simulink model "benchmark_ivan_PIANN"  (R2024b)
settings: Solver=FixedStepAuto  StartTime=0.0  StopTime=14  FixedStep=0.0001  RelTol=1e-5  AbsTol=1e-8  EnableMultiTasking=on
values from neighbouring files (symbols this model uses):
  b1 = csvread('./DAE_ANN/ANN/Biases/30_04_21/lstm_ann_pi_standard_fix_noSo4_rnn_1__100_16_b_3.csv')    [init_PI_ann.m]    (also in init_PI_ann_hier.m = csvread('./DAE_ANN/ANN/Biases/12_05_21/lstm_ann_pi_standard_; init_PI_ann_hier_v2.m = csvread('./DAE_ANN/ANN/Biases/12_05_21/lstm_ann_pi_standard_; init_PI_ann_lab.m = csvread('./DAE_ANN/ANN/Biases/12_05_21/lstm_ann_pi_standard_)
  b2 = csvread('./DAE_ANN/ANN/Biases/30_04_21/lstm_ann_pi_standard_fix_noSo4_rnn_1__100_16_b_3.csv')    [init_PI_ann.m]    (also in init_PI_ann_hier.m = csvread('./DAE_ANN/ANN/Biases/12_05_21/lstm_ann_pi_standard_; init_PI_ann_hier_v2.m = csvread('./DAE_ANN/ANN/Biases/12_05_21/lstm_ann_pi_standard_; init_PI_ann_lab.m = csvread('./DAE_ANN/ANN/Biases/12_05_21/lstm_ann_pi_standard_)
  b_last = csvread('./DAE_ANN/ANN/Biases/12_05_21/lstm_ann_pi_standard_fix_noSo4_last__100_1_b_2.csv')'    [init_PI_ann_hier.m]    (also in init_PI_ann_hier_v2.m; init_PI_ann_lab.m)
  b_out = csvread('./DAE_ANN/ANN/Biases/30_04_21/lstm_ann_pi_standard_fix_noSo4_final__100_16_b_3.csv')    [init_PI_ann.m]    (also in init_PI_ann_hier.m = csvread('./DAE_ANN/ANN/Biases/12_05_21/lstm_ann_pi_standard_; init_PI_ann_hier_v2.m = csvread('./DAE_ANN/ANN/Biases/12_05_21/lstm_ann_pi_standard_; init_PI_ann_lab.m = csvread('./DAE_ANN/ANN/Biases/12_05_21/lstm_ann_pi_standard_)
  ic_sw_Kla = 145*ones(n_sw,1)    [init_PI_ann.m]    (also in init_PI_ann_hier.m; init_PI_ann_hier_v2.m; init_PI_ann_lab.m)
  ic_sw_Snh4 = 6*ones(n_sw,1)    [init_PI_ann.m]    (also in init_PI_ann_hier.m; init_PI_ann_hier_v2.m; init_PI_ann_lab.m)
  ic_sw_Sno4 = 8*ones(n_sw,1)    [init_PI_ann.m]    (also in init_PI_ann_hier.m; init_PI_ann_hier_v2.m; init_PI_ann_lab.m)
  ic_sw_So4 = 3*ones(n_sw,1)    [init_PI_ann.m]    (also in init_PI_ann_hier.m; init_PI_ann_hier_v2.m; init_PI_ann_lab.m)
  ic_sw_So5 = 2*ones(n_sw,1)    [init_PI_ann.m]    (also in init_PI_ann_hier.m; init_PI_ann_hier_v2.m; init_PI_ann_lab.m)
  KLa5_max = 360    [sensorinit.m]
  max_Q4 = 100000    [sensorinit.m]
  max_SNH4 = 20    [sensorinit.m]
  max_SNO2 = 20    [sensorinit.m]
  max_SNO4 = 20    [sensorinit.m]
  max_SO4 = 10    [sensorinit.m]
  max_SO5 = 10    [sensorinit.m]    (also in setup_Prac5.m = 5)
  max_TSS4 = 10000    [sensorinit.m]
  mean_scaler_dir = csvread('./DAE_ANN/ANN/Scalers/30_04_21_lstm_ann_pi_standard_fix_noSo4/mean_scaler_lstm_ann_pi_standard_fix_noSo4.csv')    [init_PI_ann.m]    (also in init_PI_ann_hier.m = csvread('./DAE_ANN/ANN/Scalers/12_05_21_lstm_ann_pi_standard; init_PI_ann_hier_v2.m = csvread('./DAE_ANN/ANN/Scalers/12_05_21_lstm_ann_pi_standard; setup_Prac5.m = [(Q/k)^2, 1.9756, 0.0000, 0]')
  mean_scaler_dir_out = csvread('./DAE_ANN/ANN/Scalers/30_04_21_lstm_ann_pi_standard_fix_noSo4/mean_scaler_lstm_ann_pi_standard_fix_noSo4_out.csv')    [init_PI_ann.m]    (also in init_PI_ann_hier.m = csvread('./DAE_ANN/ANN/Scalers/12_05_21_lstm_ann_pi_standard; init_PI_ann_hier_v2.m = csvread('./DAE_ANN/ANN/Scalers/12_05_21_lstm_ann_pi_standard; setup_Prac5.m = 0)
  min_Q4 = 0    [sensorinit.m]
  min_SNH4 = 0    [sensorinit.m]
  min_SNO2 = 0    [sensorinit.m]
  min_SNO4 = 0    [sensorinit.m]
  min_SO5 = 0    [sensorinit.m]
  min_TSS4 = 0    [sensorinit.m]
  n_layers = 1    [init_PI_ann.m]    (also in init_PI_ann_hier.m; init_PI_ann_hier_v2.m; init_PI_ann_lab.m)
  n_sw = 16    [init_PI_ann.m]    (also in init_PI_ann_hier.m = 1; init_PI_ann_hier_v2.m = 1; init_PI_ann_lab.m = 1)
  n_sw_inverse = 16    [init_PI_ann.m]    (also in init_PI_ann_hier.m = 1; init_PI_ann_hier_v2.m = 1; init_PI_ann_lab.m = 1)
  noiseseed_Q4 = 1    [sensorinit.m]
  noiseseed_SNH4 = 2    [sensorinit.m]
  noiseseed_SNO2 = 2    [sensorinit.m]
  noiseseed_SNO4 = 2    [sensorinit.m]
  noiseseed_SO4 = 2    [sensorinit.m]
  noiseseed_SO5 = 1    [sensorinit.m]
  noiseseed_TSS4 = 1    [sensorinit.m]
  noisesource_Q4 = 1    [sensorinit.m]
  noisesource_SNH4 = 1    [sensorinit.m]
  noisesource_SNO2 = 1    [sensorinit.m]
  noisesource_SNO4 = 1    [sensorinit.m]
  noisesource_SO4 = 1    [sensorinit.m]
  noisesource_SO5 = 1    [sensorinit.m]
  noisesource_TSS4 = 1    [sensorinit.m]
  Qin0 = 18446    [states.mat]
  Qintr = 12141.8126939    [states.mat]
  Qintr_max = 5*Qin0    [sensorinit.m]
  Qintrawstate = 114243.527362    [states.mat]
  Qintrintstate = -116205.765277    [states.mat]
  SETTLERINIT = [12.5979803087 18.2981709885 29.6744598765 68.7829340492 352.293497132 353.981663079 351.499035887 351.323930185 355.679725774 6417.21684783 30 30 ... (80 elements, 1x80)]    [states.mat]
  Sno_mean = 1    [run_bsm1_PIANN_variable.m]
  SO5awstate = 469.399689831    [states.mat]
  SO5intstate = -450.70071346    [states.mat]
  SO5ref = 2    [run_bsm1_PIANN.m]    (also in run_bsm1_PIANN_variable.m)
  So_mean = 2    [run_bsm1_PIANN_variable.m]    (also in setup_Prac5.m = 0.2)
  std_Q4 = 0.025    [sensorinit.m]
  std_scaler_dir = csvread('./DAE_ANN/ANN/Scalers/30_04_21_lstm_ann_pi_standard_fix_noSo4/std_scaler_lstm_ann_pi_standard_fix_noSo4.csv')    [init_PI_ann.m]    (also in init_PI_ann_hier.m = csvread('./DAE_ANN/ANN/Scalers/12_05_21_lstm_ann_pi_standard; init_PI_ann_hier_v2.m = csvread('./DAE_ANN/ANN/Scalers/12_05_21_lstm_ann_pi_standard; setup_Prac5.m = [1, 0.7579, 0.05, 1]')
  std_scaler_dir_out = csvread('./DAE_ANN/ANN/Scalers/30_04_21_lstm_ann_pi_standard_fix_noSo4/std_scaler_lstm_ann_pi_standard_fix_noSo4_out.csv')    [init_PI_ann.m]    (also in init_PI_ann_hier.m = csvread('./DAE_ANN/ANN/Scalers/12_05_21_lstm_ann_pi_standard; init_PI_ann_hier_v2.m = csvread('./DAE_ANN/ANN/Scalers/12_05_21_lstm_ann_pi_standard; setup_Prac5.m = 1)
  std_SNH4 = 0.025    [sensorinit.m]
  std_SNO2 = 0.025    [sensorinit.m]
  std_SO4 = 0.025    [sensorinit.m]
  std_SO5 = 0.025    [sensorinit.m]
  std_TSS4 = 0.025    [sensorinit.m]
  T = 6.5201    [setup_Prac5.m]
  t_init = 7e-3    (= 0.007)    [run_bsm1.m]    (also in run_bsm1_PIANN_variable.m = 0.05)
  T_KLa5 = T90_KLa5/(24*60)/3.89    (= 0.000714081690945)    [sensorinit.m]
  T_Q4 = T90_Q4/(24*60)/3.89    (= 0.000178520422736)    [sensorinit.m]
  t_simulink = 1/96    (= 0.0104166666667)    [run_bsm1.m]    (also in run_bsm1_PIANN.m = -1; run_bsm1_PIANN_variable.m = 0; setup_Prac5.m = 0)
  T_SNH4 = T90_SNH4/(24*60)/11.7724    (= 0.000589891988417)    [sensorinit.m]
  T_SNO2 = T90_SNO2/(24*60)/11.7724    (= 0.000589891988417)    [sensorinit.m]
  T_SNO4 = T90_SNO4/(24*60)/11.7724    (= 0.000589891988417)    [sensorinit.m]
  T_SO5 = T90_SO5/(24*60)/3.89    (= 0.000178520422736)    [sensorinit.m]
  T_TSS4 = T90_TSS4/(24*60)/3.89    (= 0.000178520422736)    [sensorinit.m]
  t_zero_order = -1    [run_bsm1_PIANN.m]    (also in run_bsm1_PIANN_variable.m)
  u1 = csvread('./DAE_ANN/ANN/Weights/30_04_21/lstm_ann_pi_standard_fix_noSo4_rnn_1__100_16_U_3.csv')    [init_PI_ann.m]    (also in init_PI_ann_hier.m = csvread('./DAE_ANN/ANN/Weights/12_05_21/lstm_ann_pi_standard; init_PI_ann_hier_v2.m = csvread('./DAE_ANN/ANN/Weights/12_05_21/lstm_ann_pi_standard)
  u2 = csvread('./DAE_ANN/ANN/Weights/30_04_21/lstm_ann_pi_standard_fix_noSo4_rnn_1__100_16_U_3.csv')    [init_PI_ann.m]    (also in init_PI_ann_hier.m = csvread('./DAE_ANN/ANN/Weights/12_05_21/lstm_ann_pi_standard; init_PI_ann_hier_v2.m = csvread('./DAE_ANN/ANN/Weights/12_05_21/lstm_ann_pi_standard)
  useideal_KLa5 = 0    [run_bsm1.m]    (also in run_bsm1_PIANN.m = 1; run_bsm1_PIANN_variable.m = 1; sensorinit.m)
  useideal_Q4 = 1    [run_bsm1_PIANN.m]    (also in run_bsm1_PIANN_variable.m; sensorinit.m = 0)
  useideal_SNH4 = 0    [run_bsm1.m]    (also in run_bsm1_PIANN.m = 1; run_bsm1_PIANN_variable.m = 1; sensorinit.m)
  useideal_SNO2 = 1    [run_bsm1_PIANN.m]    (also in run_bsm1_PIANN_variable.m; sensorinit.m = 0)
  useideal_SNO4 = 0    [run_bsm1.m]    (also in run_bsm1_PIANN.m = 1; run_bsm1_PIANN_variable.m = 1; sensorinit.m)
  useideal_SO4 = 0    [run_bsm1.m]    (also in run_bsm1_PIANN.m = 1; run_bsm1_PIANN_variable.m = 1; sensorinit.m)
  useideal_SO5 = 0    [run_bsm1.m]    (also in run_bsm1_PIANN.m = 1; run_bsm1_PIANN_variable.m = 1; sensorinit.m)
  useideal_TSS4 = 1    [run_bsm1_PIANN.m]    (also in run_bsm1_PIANN_variable.m; sensorinit.m = 0)
  usenoise_Q4 = 0    [run_bsm1_PIANN.m]    (also in run_bsm1_PIANN_variable.m; sensorinit.m = 1)
  usenoise_SNH4 = 1    [run_bsm1.m]    (also in run_bsm1_PIANN.m = 0; run_bsm1_PIANN_variable.m = 0; sensorinit.m)
  usenoise_SNO2 = 0    [run_bsm1_PIANN.m]    (also in run_bsm1_PIANN_variable.m; sensorinit.m = 1)
  usenoise_SNO4 = 1    [run_bsm1.m]    (also in run_bsm1_PIANN.m = 0; run_bsm1_PIANN_variable.m = 0; sensorinit.m)
  usenoise_SO4 = 1    [run_bsm1.m]    (also in run_bsm1_PIANN.m = 0; run_bsm1_PIANN_variable.m = 0; sensorinit.m)
  usenoise_SO5 = 1    [run_bsm1.m]    (also in run_bsm1_PIANN.m = 0; run_bsm1_PIANN_variable.m = 0; sensorinit.m)
  usenoise_TSS4 = 0    [run_bsm1_PIANN.m]    (also in run_bsm1_PIANN_variable.m; sensorinit.m = 1)
  w1 = csvread('./DAE_ANN/ANN/Weights/30_04_21/lstm_ann_pi_standard_fix_noSo4_rnn_1__100_16_W_3.csv')    [init_PI_ann.m]    (also in init_PI_ann_hier.m = csvread('./DAE_ANN/ANN/Weights/12_05_21/lstm_ann_pi_standard; init_PI_ann_hier_v2.m = csvread('./DAE_ANN/ANN/Weights/12_05_21/lstm_ann_pi_standard; init_PI_ann_lab.m = csvread('./DAE_ANN/ANN/Weights/12_05_21/lstm_ann_pi_standard)
  w2 = csvread('./DAE_ANN/ANN/Weights/30_04_21/lstm_ann_pi_standard_fix_noSo4_rnn_1__100_16_W_3.csv')    [init_PI_ann.m]    (also in init_PI_ann_hier.m = csvread('./DAE_ANN/ANN/Weights/12_05_21/lstm_ann_pi_standard; init_PI_ann_hier_v2.m = csvread('./DAE_ANN/ANN/Weights/12_05_21/lstm_ann_pi_standard; init_PI_ann_lab.m = csvread('./DAE_ANN/ANN/Weights/12_05_21/lstm_ann_pi_standard)
  w_last = csvread('./DAE_ANN/ANN/Weights/12_05_21/lstm_ann_pi_standard_fix_noSo4_last__100_1_W_2.csv')    [init_PI_ann_hier.m]    (also in init_PI_ann_hier_v2.m; init_PI_ann_lab.m)
  w_out = csvread('./DAE_ANN/ANN/Weights/30_04_21/lstm_ann_pi_standard_fix_noSo4_final__100_16_W_3.csv')    [init_PI_ann.m]    (also in init_PI_ann_hier.m = csvread('./DAE_ANN/ANN/Weights/12_05_21/lstm_ann_pi_standard; init_PI_ann_hier_v2.m = csvread('./DAE_ANN/ANN/Weights/12_05_21/lstm_ann_pi_standard; init_PI_ann_lab.m = csvread('./DAE_ANN/ANN/Weights/12_05_21/lstm_ann_pi_standard)
  XINIT1 = [30 3.2250440682 1132.84750814 98.0848162551 2520.32093658 147.34360098 454.498440184 0.006943357113 3.54207658602 12.0720627837 1.35151294762 6.05742445882 ... (15 elements, 1x15)]    [states.mat]
  XINIT2 = [30 1.63865407136 1124.24951453 88.653599068 2501.35826654 146.001740625 452.094465666 5.17099136584e-05 1.14245691502 13.0383387996 0.796493225193 5.70045637375 ... (15 elements, 1x15)]    [states.mat]
  XINIT3 = [30 1.20592174915 1120.58961418 67.1871738861 2499.94635325 146.547839977 452.007772249 1.74081325353 6.26492922945 8.40116301472 0.827753486834 4.51387309735 ... (15 elements, 1x15)]    [states.mat]
  XINIT4 = [30 0.96656120797 1121.66055561 52.7833355811 2504.32671079 147.644975737 453.890499756 2.40137566232 11.073804945 3.99279026202 0.746788866766 3.70339113264 ... (15 elements, 1x15)]    [states.mat]
  XINIT5 = [30 0.803395489358 1124.12455116 43.2595495328 2508.23031357 148.499403125 456.322790044 2.11978031988 14.1356901459 1.15379834533 0.659650038761 3.15951382084 ... (15 elements, 1x15)]    [states.mat]
  XINITDELAY = [1466770.04249 1266021.87556 55799754.9774 5815431.95778 123179806.598 7263098.80912 22318785.5012 62039.7687555 416609.519268 588047.303413 143684.636473 343270.852984 ... (15 elements, 1x15)]    [states.mat]
undefined symbols (not defined in the file or in its folder): b_bottle, b_decoder_1, b_decoder_2, b_encoder_1, b_encoder_2, b_final, b_out_dae, carb1, carb2, carb3, carb4, carb5, DIM, Kfeedforward, KLa1, KLa2, KLa3, KLa4, KLa5offset, KQintr, KSO5, LAYER, magnitude, mean_scaler_dae, mean_scaler_dae_out, MODELTYPE, PAR1, PAR2, PAR3, PAR4, PAR5, Qffref, Qintroffset, QintrT, SETTLERPAR, SNO2ref, SOSAT1, SOSAT2, SOSAT3, SOSAT4, SOSAT5, std_scaler_dae, std_scaler_dae_out, TiQintr, TiSO5, TtQintr, TtSO5, u_decoder_1, u_decoder_2, u_encoder_1, u_encoder_2, useantiwindupQintr, useantiwindupSO5, VOL1, VOL2, VOL3, VOL4, VOL5, w_bottle, w_decoder_1 ... (+5)
libraries: dspindex x33
(part 2 of 4)

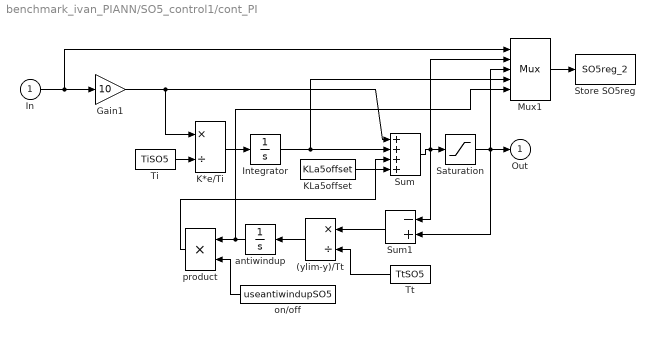
== system benchmark_ivan_PIANN/SO5_control1/cont_PI ==
  In : Inport
  (ylim-y)/Tt : Product  Inputs=*/  InputSameDT=on  SaturateOnIntegerOverflow=on  OutDataTypeStr=Inherit: Same as first input
  Gain1 : Gain  Gain=10  SaturateOnIntegerOverflow=on  OutDataTypeStr=Inherit: Same as input  ParamDataTypeStr=Inherit: Same as input
  Integrator : Integrator  InitialCondition=SO5intstate
  K*e/Ti : Product  Inputs=*/  InputSameDT=on  SaturateOnIntegerOverflow=on  OutDataTypeStr=Inherit: Same as first input
  KLa5offset : Constant  Value=KLa5offset
  Mux1 : Mux  Inputs=5
  Saturation : Saturate  UpperLimit=KLa5_max  LowerLimit=0
  Store SO5reg : ToWorkspace  VariableName=SO5reg_2  SampleTime=-1
  Sum : Sum  Inputs=++++  InputSameDT=on  SaturateOnIntegerOverflow=on  OutDataTypeStr=Inherit: Same as first input
  Sum1 : Sum  Inputs=-+  InputSameDT=on  SaturateOnIntegerOverflow=on  OutDataTypeStr=Inherit: Same as first input
  Ti : Constant  Value=TiSO5
  Tt : Constant  Value=TtSO5
  antiwindup : Integrator  InitialCondition=SO5awstate
  on/off : Constant  Value=useantiwindupSO5
  product : Product  Inputs=**  InputSameDT=on  SaturateOnIntegerOverflow=on  OutDataTypeStr=Inherit: Same as first input
  Out : Outport  VectorParamsAs1DForOutWhenUnconnected=off
  wires:
  product/1 -> Sum/3
  on/off/1 -> product/2
  K*e/Ti/1 -> Integrator/1
  Ti/1 -> K*e/Ti/2
  Gain1/1 -> Sum/1, K*e/Ti/1
  Sum1/1 -> (ylim-y)/Tt/1
  Tt/1 -> (ylim-y)/Tt/2
  (ylim-y)/Tt/1 -> antiwindup/1
  Sum/1 -> Saturation/1, Sum1/1, Mux1/2
  Saturation/1 -> Out/1, Sum1/2, Mux1/3
  Mux1/1 -> Store SO5reg/1
  Integrator/1 -> Sum/2, Mux1/4
  antiwindup/1 -> product/1, Mux1/5
  KLa5offset/1 -> Sum/4
  In/1 -> Gain1/1, Mux1/1

== system benchmark_ivan_PIANN/SO5_control_paper/Filter_Prediction ==
  Kla5 : Inport
  So5_noise : Inport  Port=2
  Measurements_1 : Inport  Port=3
  DAE_MLP1 : Subsystem  Commented=on
  DAE_MLP2 : Subsystem  Commented=on
  DAE_MLP3 : Subsystem
  DAE_lstm : Subsystem  Commented=on
  Direct Prediction LSTM4 : Subsystem
  Inverse Data : Subsystem
  Terminator : Terminator  Commented=on
  To Workspace5 : ToWorkspace  VariableName=clean_data  SampleTime=1/96
      settings: Save2DSignal=2-D array (concatenate along first dimension)
  So5_clean : Outport
  wires:
  DAE_MLP3/1(Output) -> Direct Prediction LSTM4/2(meas1), To Workspace5/1
  Inverse Data/1(Snh4) -> DAE_MLP3/1(Snh4)
  Inverse Data/2(TSS4) -> DAE_MLP3/2(TSS4)
  Inverse Data/3(Q4) -> DAE_MLP3/3(Q4)
  Kla5/1 -> Direct Prediction LSTM4/1(kla1)
  Measurements_1/1 -> Inverse Data/1(y_n1)
  Direct Prediction LSTM4/1(y_n) -> So5_clean/1
  So5_noise/1 -> DAE_MLP3/4("So5_noise ")

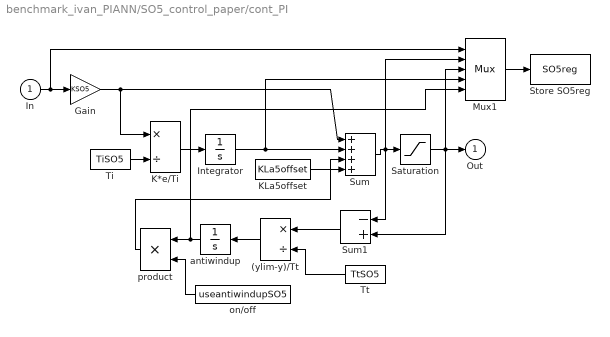
== system benchmark_ivan_PIANN/SO5_control_paper/cont_PI ==
  In : Inport
  (ylim-y)/Tt : Product  Inputs=*/  InputSameDT=on  SaturateOnIntegerOverflow=on  OutDataTypeStr=Inherit: Same as first input
  Gain : Gain  Gain=KSO5  SaturateOnIntegerOverflow=on  OutDataTypeStr=Inherit: Same as input  ParamDataTypeStr=Inherit: Same as input
  Integrator : Integrator  InitialCondition=SO5intstate
  K*e/Ti : Product  Inputs=*/  InputSameDT=on  SaturateOnIntegerOverflow=on  OutDataTypeStr=Inherit: Same as first input
  KLa5offset : Constant  Value=KLa5offset
  Mux1 : Mux  Inputs=5
  Saturation : Saturate  UpperLimit=KLa5_max  LowerLimit=0
  Store SO5reg : ToWorkspace  VariableName=SO5reg  SampleTime=-1
  Sum : Sum  Inputs=++++  InputSameDT=on  SaturateOnIntegerOverflow=on  OutDataTypeStr=Inherit: Same as first input
  Sum1 : Sum  Inputs=-+  InputSameDT=on  SaturateOnIntegerOverflow=on  OutDataTypeStr=Inherit: Same as first input
  Ti : Constant  Value=TiSO5
  Tt : Constant  Value=TtSO5
  antiwindup : Integrator  InitialCondition=SO5awstate
  on/off : Constant  Value=useantiwindupSO5
  product : Product  Inputs=**  InputSameDT=on  SaturateOnIntegerOverflow=on  OutDataTypeStr=Inherit: Same as first input
  Out : Outport  VectorParamsAs1DForOutWhenUnconnected=off
  wires:
  product/1 -> Sum/3
  on/off/1 -> product/2
  In/1 -> Mux1/1, Gain/1
  K*e/Ti/1 -> Integrator/1
  Ti/1 -> K*e/Ti/2
  Gain/1 -> Sum/1, K*e/Ti/1
  Sum1/1 -> (ylim-y)/Tt/1
  Tt/1 -> (ylim-y)/Tt/2
  (ylim-y)/Tt/1 -> antiwindup/1
  Sum/1 -> Saturation/1, Sum1/1, Mux1/2
  Saturation/1 -> Out/1, Sum1/2, Mux1/3
  Mux1/1 -> Store SO5reg/1
  Integrator/1 -> Sum/2, Mux1/4
  antiwindup/1 -> product/1, Mux1/5
  KLa5offset/1 -> Sum/4

== system benchmark_ivan_PIANN/Direct Prediction 2 LSTM SO1/Data Preprocesing Direct/Normalizer1 ==
  Data Input : Inport
  Normalization Values : MATLAB Function  TreatAsAtomicUnit=on
  Data Normalized : Outport  VectorParamsAs1DForOutWhenUnconnected=off
  wires:
  Data Input/1 -> Normalization Values/1(data_input)
  Normalization Values/1(data_norm) -> Data Normalized/1

== system benchmark_ivan_PIANN/Direct Prediction 2 LSTM SO1/Sliding Window/Sliding Window Buffer So1 ==
  In1 : Inport
  Buffer1 : Buffer  N=16  V=15
  Reshape : Reshape
  Zero-Order Hold : ZeroOrderHold  SampleTime=1/96
  Out1 : Outport
  wires:
  Zero-Order Hold/1 -> Buffer1/1
  In1/1 -> Zero-Order Hold/1
  Reshape/1 -> Out1/1
  Buffer1/1 -> Reshape/1

== system benchmark_ivan_PIANN/Direct Prediction 2 LSTM SO1/Sliding Window/Sliding Window Buffer So2 ==
  In1 : Inport
  Buffer1 : Buffer  N=16  V=15
  Reshape : Reshape
  Zero-Order Hold : ZeroOrderHold  SampleTime=1/96
  Out1 : Outport
  wires:
  Zero-Order Hold/1 -> Buffer1/1
  In1/1 -> Zero-Order Hold/1
  Reshape/1 -> Out1/1
  Buffer1/1 -> Reshape/1

== system benchmark_ivan_PIANN/Direct Prediction 2 LSTM SO1/Sliding Window/Sliding Window Buffer So3 ==
  In1 : Inport
  Buffer1 : Buffer  N=16  V=15
  Reshape : Reshape
  Zero-Order Hold : ZeroOrderHold  SampleTime=-1
  Out1 : Outport
  wires:
  Zero-Order Hold/1 -> Buffer1/1
  In1/1 -> Zero-Order Hold/1
  Reshape/1 -> Out1/1
  Buffer1/1 -> Reshape/1

== system benchmark_ivan_PIANN/Direct Prediction 2 LSTM SO1/Sliding Window/Sliding Window Buffer So4 ==
  In1 : Inport
  Buffer1 : Buffer  N=16  V=15
  Reshape : Reshape
  Zero-Order Hold : ZeroOrderHold  SampleTime=1/96
  Out1 : Outport
  wires:
  Zero-Order Hold/1 -> Buffer1/1
  In1/1 -> Zero-Order Hold/1
  Reshape/1 -> Out1/1
  Buffer1/1 -> Reshape/1

== system benchmark_ivan_PIANN/Direct Prediction LSTM3/Data Preprocesing Direct/Normalizer1 ==
  Data Input : Inport
  Normalization Values : MATLAB Function  TreatAsAtomicUnit=on
  Data Normalized : Outport  VectorParamsAs1DForOutWhenUnconnected=off
  wires:
  Normalization Values/1(data_norm) -> Data Normalized/1
  Data Input/1 -> Normalization Values/1(data_input)

== system benchmark_ivan_PIANN/Direct Prediction LSTM3/Sliding Window/Sliding Window Buffer So1 ==
  In1 : Inport
  Buffer1 : Buffer  N=16  V=15
  Reshape : Reshape
  Zero-Order Hold : ZeroOrderHold  SampleTime=1/96
  Out1 : Outport
  wires:
  Buffer1/1 -> Reshape/1
  Reshape/1 -> Out1/1
  In1/1 -> Zero-Order Hold/1
  Zero-Order Hold/1 -> Buffer1/1

== system benchmark_ivan_PIANN/Direct Prediction LSTM3/Sliding Window/Sliding Window Buffer So2 ==
  In1 : Inport
  Buffer1 : Buffer  N=16  V=15
  Reshape : Reshape
  Zero-Order Hold : ZeroOrderHold  SampleTime=1/96
  Out1 : Outport
  wires:
  Buffer1/1 -> Reshape/1
  Reshape/1 -> Out1/1
  In1/1 -> Zero-Order Hold/1
  Zero-Order Hold/1 -> Buffer1/1

== system benchmark_ivan_PIANN/Direct Prediction LSTM3/Sliding Window/Sliding Window Buffer So3 ==
  In1 : Inport
  Buffer1 : Buffer  N=16  V=15
  Reshape : Reshape
  Zero-Order Hold : ZeroOrderHold  SampleTime=-1
  Out1 : Outport
  wires:
  Buffer1/1 -> Reshape/1
  Reshape/1 -> Out1/1
  In1/1 -> Zero-Order Hold/1
  Zero-Order Hold/1 -> Buffer1/1

== system benchmark_ivan_PIANN/Direct Prediction LSTM3/Sliding Window/Sliding Window Buffer So4 ==
  In1 : Inport
  Buffer1 : Buffer  N=16  V=15
  Reshape : Reshape
  Zero-Order Hold : ZeroOrderHold  SampleTime=1/96
  Out1 : Outport
  wires:
  Buffer1/1 -> Reshape/1
  Reshape/1 -> Out1/1
  In1/1 -> Zero-Order Hold/1
  Zero-Order Hold/1 -> Buffer1/1

== system benchmark_ivan_PIANN/Direct Prediction LSTM3/Sliding Window/Sliding Window1 ==
  ref1 : Inport
  Delay : Delay  DelayLength=1  InitialCondition=0  SampleTime=t_simulink
  Flip : DSPFlip
  IC : InitialCondition  Value=zeros(16,1)
  Mux : Mux  Inputs=2
  Variable Selector : dspindex/Variable Selector  NumInputs=1  rowsOrCols=Rows  IdxMode=Fixed  Elements=1:15  ZerOneIdxMode=One-based  errmode=Clip Index  FillMode=on  FillValues=0
  Out : Outport
  wires:
  IC/1 -> Variable Selector/1
  Delay/1 -> IC/1
  ref1/1 -> Mux/1
  Variable Selector/1 -> Mux/2
  Flip/1 -> Out/1
  Mux/1 -> Delay/1, Flip/1

== system benchmark_ivan_PIANN/Direct Prediction LSTM3/Sliding Window/Sliding Window2 ==
  data : Inport
  Delay : Delay  DelayLength=1  InitialCondition=0  SampleTime=t_simulink
  Flip : DSPFlip
  IC : InitialCondition  Value=zeros(16,1)
  Mux : Mux  Inputs=2
  Variable Selector : dspindex/Variable Selector  NumInputs=1  rowsOrCols=Rows  IdxMode=Fixed  Elements=1:15  ZerOneIdxMode=One-based  errmode=Clip Index  FillMode=on  FillValues=0
  Out : Outport
  wires:
  IC/1 -> Variable Selector/1
  Delay/1 -> IC/1
  data/1 -> Mux/1
  Variable Selector/1 -> Mux/2
  Flip/1 -> Out/1
  Mux/1 -> Delay/1, Flip/1

== system benchmark_ivan_PIANN/Direct Prediction LSTM3/Sliding Window/Sliding Window3 ==
  ref : Inport
  Delay : Delay  DelayLength=1  InitialCondition=0  SampleTime=t_simulink
  Flip : DSPFlip
  IC : InitialCondition  Value=zeros(16,1)
  Mux : Mux  Inputs=2
  Variable Selector : dspindex/Variable Selector  NumInputs=1  rowsOrCols=Rows  IdxMode=Fixed  Elements=1:15  ZerOneIdxMode=One-based  errmode=Clip Index  FillMode=on  FillValues=0
  Out : Outport
  wires:
  IC/1 -> Variable Selector/1
  Delay/1 -> IC/1
  ref/1 -> Mux/1
  Variable Selector/1 -> Mux/2
  Flip/1 -> Out/1
  Mux/1 -> Delay/1, Flip/1

== system benchmark_ivan_PIANN/Direct Prediction LSTM3/Sliding Window/Sliding Window4 ==
  delayed : Inport
  Delay : Delay  DelayLength=1  InitialCondition=0  SampleTime=t_simulink
  Flip : DSPFlip
  IC : InitialCondition  Value=zeros(16,1)
  Mux : Mux  Inputs=2
  Variable Selector : dspindex/Variable Selector  NumInputs=1  rowsOrCols=Rows  IdxMode=Fixed  Elements=1:15  ZerOneIdxMode=One-based  errmode=Clip Index  FillMode=on  FillValues=0
  Out : Outport
  wires:
  IC/1 -> Variable Selector/1
  Delay/1 -> IC/1
  delayed/1 -> Mux/1
  Variable Selector/1 -> Mux/2
  Flip/1 -> Out/1
  Mux/1 -> Delay/1, Flip/1

== system benchmark_ivan_PIANN/Direct Prediction LSTM3/Sliding Window/Sliding Window6 ==
  ref1 : Inport
  Delay : Delay  DelayLength=1  InitialCondition=0  SampleTime=t_simulink
  Flip : DSPFlip
  IC : InitialCondition  Value=zeros(16,1)
  Mux : Mux  Inputs=2
  Variable Selector : dspindex/Variable Selector  NumInputs=1  rowsOrCols=Rows  IdxMode=Fixed  Elements=1:15  ZerOneIdxMode=One-based  errmode=Clip Index  FillMode=on  FillValues=0
  Out : Outport
  wires:
  IC/1 -> Variable Selector/1
  Delay/1 -> IC/1
  ref1/1 -> Mux/1
  Variable Selector/1 -> Mux/2
  Flip/1 -> Out/1
  Mux/1 -> Delay/1, Flip/1

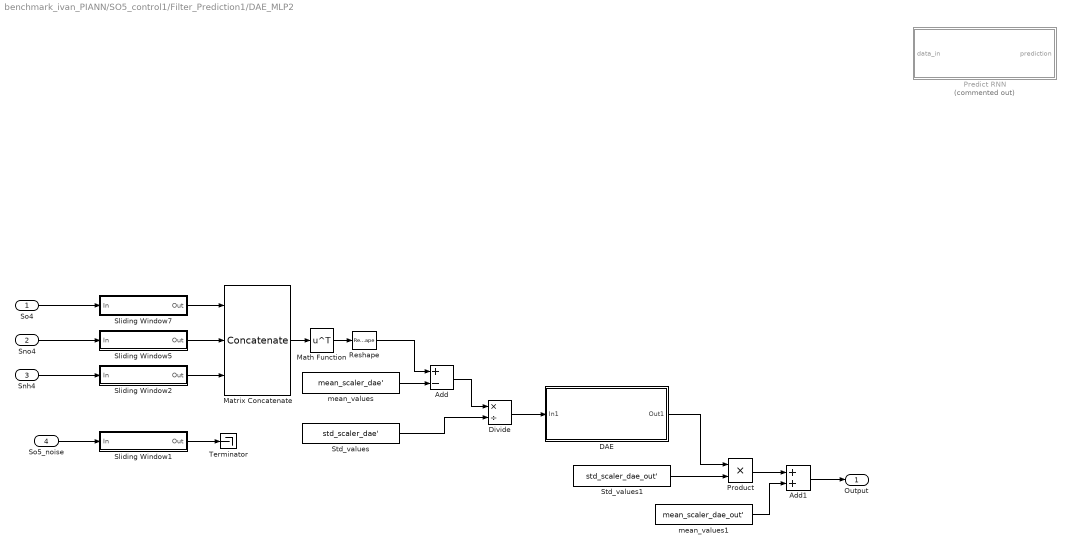
== system benchmark_ivan_PIANN/SO5_control1/Filter_Prediction1/DAE_MLP2 ==
  So4 : Inport
  Sno4 : Inport  Port=2
  Snh4 : Inport  Port=3
  "So5_noise " : Inport  Port=4
  Add : Sum  Inputs=+-
  Add1 : Sum
  DAE : Subsystem
  Divide : Product  Inputs=*/
  Math Function : Math  Operator=transpose  SignedPower=on
  Matrix Concatenate : Concatenate  NumInputs=3  Mode=Multidimensional array  ConcatenateDimension=2
  Predict RNN : MATLAB Function  Commented=on  TreatAsAtomicUnit=on
  Product : Product
  Reshape : Reshape  OutputDimensionality=Row vector (2-D)
  Sliding Window1 : Subsystem
  Sliding Window2 : Subsystem
  Sliding Window5 : Subsystem
  Sliding Window7 : Subsystem
  Std_values : Constant  Value=std_scaler_dae'  VectorParams1D=off
  Std_values1 : Constant  Value=std_scaler_dae_out'  VectorParams1D=off
  Terminator : Terminator
  mean_values : Constant  Value=mean_scaler_dae'  VectorParams1D=off
  mean_values1 : Constant  Value=mean_scaler_dae_out'  VectorParams1D=off
  Output : Outport  VectorParamsAs1DForOutWhenUnconnected=off
  wires:
  Add1/1 -> Output/1
  Sliding Window7/1(Out) -> Matrix Concatenate/1
  Math Function/1 -> Reshape/1
  Matrix Concatenate/1 -> Math Function/1
  Sliding Window1/1(Out) -> Terminator/1
  "So5_noise "/1 -> Sliding Window1/1(In)
  Sliding Window5/1(Out) -> Matrix Concatenate/2
  Sliding Window2/1(Out) -> Matrix Concatenate/3
  Sno4/1 -> Sliding Window5/1(In)
  So4/1 -> Sliding Window7/1(In)
  Snh4/1 -> Sliding Window2/1(In)
  Add/1 -> Divide/1
  Std_values/1 -> Divide/2
  mean_values/1 -> Add/2
  Reshape/1 -> Add/1
  Divide/1 -> DAE/1(In1)
  DAE/1(Out1) -> Product/1
  Std_values1/1 -> Product/2
  Product/1 -> Add1/1
  mean_values1/1 -> Add1/2

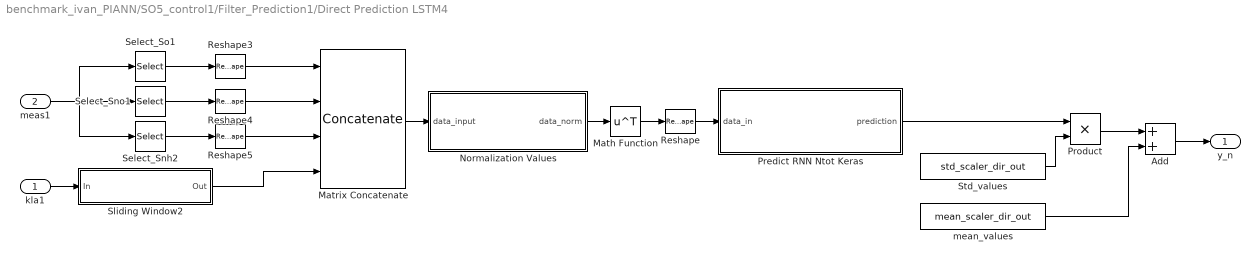
== system benchmark_ivan_PIANN/SO5_control1/Filter_Prediction1/Direct Prediction LSTM4 ==
  kla1 : Inport
  meas1 : Inport  Port=2
  Add : Sum
  Math Function : Math  Operator=transpose  SignedPower=on
  Matrix Concatenate : Concatenate  NumInputs=4  Mode=Multidimensional array  ConcatenateDimension=2
  Normalization Values : MATLAB Function  TreatAsAtomicUnit=on
  Predict RNN Ntot Keras : MATLAB Function  TreatAsAtomicUnit=on
  Product : Product
  Reshape : Reshape  OutputDimensionality=Row vector (2-D)
  Reshape3 : Reshape
  Reshape4 : Reshape
  Reshape5 : Reshape
  Select_Snh2 : Selector  NumberOfDimensions=2  InputPortWidth=4  IndexOptions=Index vector (dialog),Index vector (dialog)  Indices=1,[3:3:48]  OutputSizes=1,1
  Select_Sno1 : Selector  NumberOfDimensions=2  InputPortWidth=4  IndexOptions=Index vector (dialog),Index vector (dialog)  Indices=1,[2:3:48]  OutputSizes=1,1
  Select_So1 : Selector  NumberOfDimensions=2  InputPortWidth=4  IndexOptions=Index vector (dialog),Index vector (dialog)  Indices=1,[1:3:48]  OutputSizes=1,1
  Sliding Window2 : Subsystem
  Std_values : Constant  Value=std_scaler_dir_out  VectorParams1D=off
  mean_values : Constant  Value=mean_scaler_dir_out  VectorParams1D=off
  y_n : Outport  VectorParamsAs1DForOutWhenUnconnected=off
  wires:
  Reshape/1 -> Predict RNN Ntot Keras/1(data_in)
  Add/1 -> y_n/1
  Product/1 -> Add/1
  mean_values/1 -> Add/2
  Predict RNN Ntot Keras/1(prediction) -> Product/1
  Std_values/1 -> Product/2
  Math Function/1 -> Reshape/1
  Matrix Concatenate/1 -> Normalization Values/1(data_input)
  Normalization Values/1(data_norm) -> Math Function/1
  Sliding Window2/1(Out) -> Matrix Concatenate/4
  Reshape3/1 -> Matrix Concatenate/1
  Select_Sno1/1 -> Reshape4/1
  kla1/1 -> Sliding Window2/1(In)
  Reshape4/1 -> Matrix Concatenate/2
  Reshape5/1 -> Matrix Concatenate/3
  Select_Snh2/1 -> Reshape5/1
  Select_So1/1 -> Reshape3/1
  meas1/1 -> Select_Sno1/1, Select_Snh2/1, Select_So1/1

== system benchmark_ivan_PIANN/SO5_control1/Filter_Prediction1/SNH4_sensor_(B0) ==
  note: SENSOR CLASS: B0
  u : Inport
  Constant : Constant  Value=usenoise_SNH4
  Constant1 : Constant  Value=noisesource_SNH4
  Constant2 : Constant  Value=useideal_SNH4
  From Workspace : FromWorkspace  VariableName=NOISEDATA_SNH4  ZeroCross=off
  Gain : Gain  Gain=max_SNH4*std_SNH4  SaturateOnIntegerOverflow=on  OutDataTypeStr=Inherit: Same as input  ParamDataTypeStr=Inherit: Same as input
  Mux : Mux  Inputs=6
  Product : Product  InputSameDT=on  SaturateOnIntegerOverflow=on  OutDataTypeStr=Inherit: Same as first input
  Random Number : RandomNumber  Seed=noiseseed_SNH4  SampleTime=1/1440
  Saturation : Saturate  UpperLimit=max_SNH4  LowerLimit=min_SNH4
  Select_SNO : Selector  InputPortWidth=15  IndexOptions=Index vector (dialog)  Indices=[10]  OutputSizes=1
  Sum : Sum  Inputs=|++  InputSameDT=on  SaturateOnIntegerOverflow=on  OutDataTypeStr=Inherit: Same as first input
  Switch : Switch  Threshold=0.5  SaturateOnIntegerOverflow=off  InputSameDT=off
  Switch1 : Switch  Threshold=0.5  SaturateOnIntegerOverflow=off  InputSameDT=off
  To Workspace : ToWorkspace  VariableName=SNH4sensor  SampleTime=-1
  eight order Laplace : TransferFcn  Denominator=[ T_SNH4*T_SNH4*T_SNH4*T_SNH4*T_SNH4*T_SNH4*T_SNH4*T_SNH4, 8*T_SNH4*T_SNH4*T_SNH4*T_SNH4*T_SNH4*T_SNH4*T_SNH4, 28*T_SNH4*T_SNH4*T_SNH4*T_SNH4*T_SNH4*T_SNH4, 56*T_SNH4*T_SNH4*T_SNH4*T_SNH4*T_SNH4, 70*T_SNH4*T_SNH4*T_SNH4*T_SNH4, 56*T_SNH4*T_SNH4*T_SNH4, 28*T_SNH4*T_SNH4, 8* T_SNH4, 1]
  y : Outport  VectorParamsAs1DForOutWhenUnconnected=off
  wires:
  Mux/1 -> To Workspace/1
  Constant2/1 -> Switch1/2
  Switch1/1 -> Mux/6, y/1
  Saturation/1 -> Switch1/3
  Random Number/1 -> Switch/3
  Constant1/1 -> Switch/2
  From Workspace/1 -> Switch/1
  Constant/1 -> Product/1
  Switch/1 -> Gain/1
  Gain/1 -> Product/2
  Select_SNO/1 -> Mux/1, Switch1/1, eight order Laplace/1
  u/1 -> Select_SNO/1
  Product/1 -> Mux/4, Sum/2
  eight order Laplace/1 -> Mux/3, Mux/2, Sum/1
  Sum/1 -> Mux/5, Saturation/1

== system benchmark_ivan_PIANN/SO5_control1/Filter_Prediction1/SNO4_sensor_(B0) ==
  note: SENSOR CLASS: B0
  u : Inport
  Constant : Constant  Value=usenoise_SNO4
  Constant1 : Constant  Value=noisesource_SNO4
  Constant2 : Constant  Value=useideal_SNO4
  From Workspace : FromWorkspace  VariableName=NOISEDATA_SNO4  ZeroCross=off
  Gain : Gain  Gain=max_SNO2*std_SNO2  SaturateOnIntegerOverflow=on  OutDataTypeStr=Inherit: Same as input  ParamDataTypeStr=Inherit: Same as input
  Mux : Mux  Inputs=6
  Product : Product  InputSameDT=on  SaturateOnIntegerOverflow=on  OutDataTypeStr=Inherit: Same as first input
  Random Number : RandomNumber  Seed=noiseseed_SNO4  SampleTime=1/1440
  Saturation : Saturate  UpperLimit=max_SNO4  LowerLimit=min_SNO4
  Select_SNO : Selector  InputPortWidth=15  IndexOptions=Index vector (dialog)  Indices=[9]  OutputSizes=1
  Sum : Sum  Inputs=|++  InputSameDT=on  SaturateOnIntegerOverflow=on  OutDataTypeStr=Inherit: Same as first input
  Switch : Switch  Threshold=0.5  SaturateOnIntegerOverflow=off  InputSameDT=off
  Switch1 : Switch  Threshold=0.5  SaturateOnIntegerOverflow=off  InputSameDT=off
  To Workspace : ToWorkspace  VariableName=SNO4sensor  SampleTime=-1
  eight order Laplace : TransferFcn  Denominator=[ T_SNO4*T_SNO4*T_SNO4*T_SNO4*T_SNO4*T_SNO4*T_SNO4*T_SNO4, 8*T_SNO4*T_SNO4*T_SNO4*T_SNO4*T_SNO4*T_SNO4*T_SNO4, 28*T_SNO4*T_SNO4*T_SNO4*T_SNO4*T_SNO4*T_SNO4, 56*T_SNO4*T_SNO4*T_SNO4*T_SNO4*T_SNO4, 70*T_SNO4*T_SNO4*T_SNO4*T_SNO4, 56*T_SNO4*T_SNO4*T_SNO4, 28*T_SNO4*T_SNO4, 8* T_SNO4, 1]
  y : Outport  VectorParamsAs1DForOutWhenUnconnected=off
  wires:
  Mux/1 -> To Workspace/1
  Constant2/1 -> Switch1/2
  Switch1/1 -> Mux/6, y/1
  Saturation/1 -> Switch1/3
  Random Number/1 -> Switch/3
  Constant1/1 -> Switch/2
  From Workspace/1 -> Switch/1
  Constant/1 -> Product/1
  Switch/1 -> Gain/1
  Gain/1 -> Product/2
  Select_SNO/1 -> Mux/1, Switch1/1, eight order Laplace/1
  u/1 -> Select_SNO/1
  Product/1 -> Mux/4, Sum/2
  eight order Laplace/1 -> Mux/3, Mux/2, Sum/1
  Sum/1 -> Mux/5, Saturation/1

== system benchmark_ivan_PIANN/SO5_control1/Filter_Prediction1/SO4_sensor_(A) ==
  note: SENSOR CLASS: A
  u : Inport
  Constant : Constant  Value=usenoise_SO4
  Constant1 : Constant  Value=noisesource_SO4
  Constant2 : Constant  Value=useideal_SO4
  From Workspace : FromWorkspace  VariableName=NOISEDATA_SO4  ZeroCross=off
  Gain : Gain  Gain=max_SO4*std_SO4  SaturateOnIntegerOverflow=on  OutDataTypeStr=Inherit: Same as input  ParamDataTypeStr=Inherit: Same as input
  Mux : Mux  Inputs=6
  Product : Product  InputSameDT=on  SaturateOnIntegerOverflow=on  OutDataTypeStr=Inherit: Same as first input
  Random Number : RandomNumber  Seed=noiseseed_SO4  SampleTime=1/1440
  Saturation : Saturate  UpperLimit=max_SO5  LowerLimit=min_SO5
  Select_DO : Selector  InputPortWidth=15  IndexOptions=Index vector (dialog)  Indices=[8]  OutputSizes=1
  Sum : Sum  Inputs=|++  InputSameDT=on  SaturateOnIntegerOverflow=on  OutDataTypeStr=Inherit: Same as first input
  Switch : Switch  Threshold=0.5  SaturateOnIntegerOverflow=off  InputSameDT=off
  Switch1 : Switch  Threshold=0.5  SaturateOnIntegerOverflow=off  InputSameDT=off
  To Workspace : ToWorkspace  VariableName=SO4sensor  SampleTime=-1
  second order Laplace : TransferFcn  Denominator=[ T_SO5*T_SO5, 2*T_SO5, 1]
  y : Outport  VectorParamsAs1DForOutWhenUnconnected=off
  wires:
  Mux/1 -> To Workspace/1
  Constant2/1 -> Switch1/2
  Switch1/1 -> Mux/6, y/1
  Saturation/1 -> Switch1/3
  Random Number/1 -> Switch/3
  Constant1/1 -> Switch/2
  From Workspace/1 -> Switch/1
  Constant/1 -> Product/1
  Switch/1 -> Gain/1
  Gain/1 -> Product/2
  Select_DO/1 -> Mux/1, Switch1/1, second order Laplace/1
  u/1 -> Select_DO/1
  Product/1 -> Mux/4, Sum/2
  second order Laplace/1 -> Mux/3, Mux/2, Sum/1
  Sum/1 -> Mux/5, Saturation/1

== system benchmark_ivan_PIANN/SO5_control_paper/Filter_Prediction/DAE_MLP1 ==
  So4 : Inport
  Sno4 : Inport  Port=2
  Snh4 : Inport  Port=3
  DAE : Subsystem
  Data Preprocesing Direct : Subsystem
  Data Preprocessing Direct1 : Subsystem
  Sliding Window : Subsystem
  Output : Outport  VectorParamsAs1DForOutWhenUnconnected=off
  wires:
  Data Preprocesing Direct/1(Out1) -> DAE/1(x_norm)
  Sliding Window/1(Out1) -> Data Preprocesing Direct/1(u_n)
  DAE/1(y_n) -> Data Preprocessing Direct1/1(y_n)
  So4/1 -> Sliding Window/1(So4)
  Data Preprocessing Direct1/1(Out1) -> Output/1
  Sno4/1 -> Sliding Window/2(Sno4)
  Snh4/1 -> Sliding Window/3(Snh4)

== system benchmark_ivan_PIANN/SO5_control_paper/Filter_Prediction/DAE_MLP2 ==
  So4 : Inport
  Sno4 : Inport  Port=2
  Snh4 : Inport  Port=3
  "So5_noise " : Inport  Port=4
  DAE : Subsystem
  Data Preprocesing Direct : Subsystem
  Data Preprocessing Direct1 : Subsystem
  Sliding Window : Subsystem
  Output : Outport  VectorParamsAs1DForOutWhenUnconnected=off
  wires:
  Data Preprocesing Direct/1(Out1) -> DAE/1(x_norm)
  Sliding Window/1(Out1) -> Data Preprocesing Direct/1(u_n)
  DAE/1(y_n) -> Data Preprocessing Direct1/1(y_n)
  So4/1 -> Sliding Window/1(So4)
  Data Preprocessing Direct1/1(Out1) -> Output/1
  "So5_noise "/1 -> Sliding Window/4(So5)
  Snh4/1 -> Sliding Window/3(Snh4)
  Sno4/1 -> Sliding Window/2(Sno4)

== system benchmark_ivan_PIANN/SO5_control_paper/Filter_Prediction/DAE_MLP3 ==
  Snh4 : Inport
  TSS4 : Inport  Port=2
  Q4 : Inport  Port=3
  "So5_noise " : Inport  Port=4
  DAE : Subsystem
  Data Preprocesing Direct : Subsystem
  Data Preprocessing Direct1 : Subsystem
  Sliding Window : Subsystem
  Output : Outport  VectorParamsAs1DForOutWhenUnconnected=off
  wires:
  Data Preprocesing Direct/1(Out1) -> DAE/1(x_norm)
  Sliding Window/1(Out1) -> Data Preprocesing Direct/1(u_n)
  DAE/1(y_n) -> Data Preprocessing Direct1/1(y_n)
  Snh4/1 -> Sliding Window/1(Snh4)
  Data Preprocessing Direct1/1(Out1) -> Output/1
  TSS4/1 -> Sliding Window/3(TSS4)
  Q4/1 -> Sliding Window/4(Q4)
  "So5_noise "/1 -> Sliding Window/2(So5)

== system benchmark_ivan_PIANN/SO5_control_paper/Filter_Prediction/DAE_lstm ==
  So4 : Inport
  Sno4 : Inport  Port=2
  Snh4 : Inport  Port=3
  So5 : Inport  Port=4
  DAE : Subsystem
  Data Preprocesing Direct : Subsystem
  Data Preprocessing Direct1 : Subsystem
  MATLAB Function : MATLAB Function  Commented=on  TreatAsAtomicUnit=on
  Sliding Window : Subsystem
  Output : Outport  VectorParamsAs1DForOutWhenUnconnected=off
  wires:
  Data Preprocesing Direct/1(Out1) -> DAE/1(x_norm)
  DAE/1(y_n) -> Data Preprocessing Direct1/1(y_n)
  Sliding Window/1(Out1) -> Data Preprocesing Direct/1(u_n)
  Data Preprocessing Direct1/1(Out1) -> Output/1
  So4/1 -> Sliding Window/1(So4)
  Sno4/1 -> Sliding Window/2(Sno4)
  Snh4/1 -> Sliding Window/3(Snh4)
  So5/1 -> Sliding Window/4(So5)

== system benchmark_ivan_PIANN/SO5_control_paper/Filter_Prediction/Direct Prediction LSTM4 ==
  kla1 : Inport
  meas1 : Inport  Port=2
  Data Preprocesing Direct : Subsystem
  Data Preprocessing Direct1 : Subsystem
  Direct ANN : Subsystem
  Saturation : Saturate  UpperLimit=max_SO5  LowerLimit=0
  Sliding Window 1 : Subsystem
  "Sliding Window 48 " : Subsystem  Commented=on
  Sliding Window 64 : Subsystem  Commented=on
  Sliding Window 64 with So5 : Subsystem  Commented=on
  Zero-Order Hold2 : ZeroOrderHold  Commented=on  SampleTime=t_zero_order
  y_n : Outport  VectorParamsAs1DForOutWhenUnconnected=off
  wires:
  Data Preprocesing Direct/1(Out1) -> Direct ANN/1(x_norm)
  Direct ANN/1(y_n) -> Data Preprocessing Direct1/1(y_n)
  Data Preprocessing Direct1/1(Out1) -> Saturation/1
  Sliding Window 1/1(Out1) -> Data Preprocesing Direct/1(u_n)
  meas1/1 -> Sliding Window 1/1(data1)
  kla1/1 -> Sliding Window 1/2(ref)
  Saturation/1 -> y_n/1

== system benchmark_ivan_PIANN/SO5_control_paper/Filter_Prediction/Inverse Data ==
  y_n1 : Inport
  " Q4_sensor_(A)" : Subsystem
  SNH4_sensor_(B0) : Subsystem
  TSS4_sensor_(A) : Subsystem
  Snh4 : Outport  VectorParamsAs1DForOutWhenUnconnected=off
  TSS4 : Outport  Port=2  VectorParamsAs1DForOutWhenUnconnected=off
  Q4 : Outport  Port=3  VectorParamsAs1DForOutWhenUnconnected=off
  wires:
  y_n1/1 -> " Q4_sensor_(A)"/1(u), TSS4_sensor_(A)/1(u), SNH4_sensor_(B0)/1(u)
  SNH4_sensor_(B0)/1(y) -> Snh4/1
  TSS4_sensor_(A)/1(y) -> TSS4/1
  " Q4_sensor_(A)"/1(y) -> Q4/1

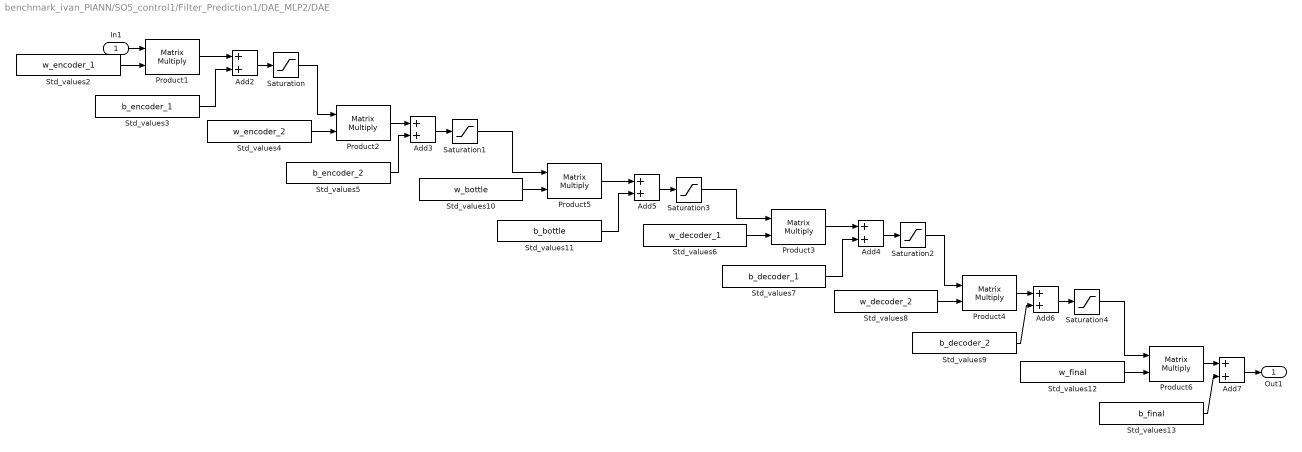
== system benchmark_ivan_PIANN/SO5_control1/Filter_Prediction1/DAE_MLP2/DAE ==
  In1 : Inport
  Add{2..7} (6 alike) : Sum
  Product{1..6} (6 alike) : Product  Multiplication=Matrix(*)
  Saturation{,1..4} (5 alike) : Saturate  UpperLimit=inf  LowerLimit=0
  Std_values10 : Constant  Value=w_bottle  VectorParams1D=off
  Std_values11 : Constant  Value=b_bottle  VectorParams1D=off
  Std_values12 : Constant  Value=w_final  VectorParams1D=off
  Std_values13 : Constant  Value=b_final  VectorParams1D=off
  Std_values2 : Constant  Value=w_encoder_1  VectorParams1D=off
  Std_values3 : Constant  Value=b_encoder_1  VectorParams1D=off
  Std_values4 : Constant  Value=w_encoder_2  VectorParams1D=off
  Std_values5 : Constant  Value=b_encoder_2  VectorParams1D=off
  Std_values6 : Constant  Value=w_decoder_1  VectorParams1D=off
  Std_values7 : Constant  Value=b_decoder_1  VectorParams1D=off
  Std_values8 : Constant  Value=w_decoder_2  VectorParams1D=off
  Std_values9 : Constant  Value=b_decoder_2  VectorParams1D=off
  Out1 : Outport
  wires:
  Std_values5/1 -> Add3/2
  Saturation4/1 -> Product6/1
  Product5/1 -> Add5/1
  Std_values11/1 -> Add5/2
  Add2/1 -> Saturation/1
  Product3/1 -> Add4/1
  Saturation1/1 -> Product5/1
  Std_values12/1 -> Product6/2
  Product2/1 -> Add3/1
  In1/1 -> Product1/1
  Std_values9/1 -> Add6/2
  Add7/1 -> Out1/1
  Add3/1 -> Saturation1/1
  Std_values7/1 -> Add4/2
  Saturation2/1 -> Product4/1
  Std_values4/1 -> Product2/2
  Product4/1 -> Add6/1
  Std_values2/1 -> Product1/2
  Saturation3/1 -> Product3/1
  Std_values6/1 -> Product3/2
  Std_values3/1 -> Add2/2
  Saturation/1 -> Product2/1
  Std_values8/1 -> Product4/2
  Add5/1 -> Saturation3/1
  Std_values13/1 -> Add7/2
  Product1/1 -> Add2/1
  Add6/1 -> Saturation4/1
  Add4/1 -> Saturation2/1
  Product6/1 -> Add7/1
  Std_values10/1 -> Product5/2

== system benchmark_ivan_PIANN/SO5_control1/Filter_Prediction1/DAE_MLP2/Sliding Window1 ==
  In : Inport
  Delay1 : Delay  DelayLength=1  InitialCondition=2  SampleTime=t_simulink
  Flip : DSPFlip
  IC : InitialCondition  Value=ic_sw_So5
  Mux : Mux  Inputs=2
  To Workspace5 : ToWorkspace  VariableName=sw_So5  SampleTime=1/96
  Variable Selector : dspindex/Variable Selector  NumInputs=1  rowsOrCols=Rows  IdxMode=Fixed  Elements=1:(n_sw_inverse-1)  ZerOneIdxMode=One-based  errmode=Clip Index  FillMode=on  FillValues=0
  Out : Outport  VectorParamsAs1DForOutWhenUnconnected=off
  wires:
  IC/1 -> Variable Selector/1
  Delay1/1 -> IC/1
  In/1 -> Mux/1
  Variable Selector/1 -> Mux/2
  Flip/1 -> To Workspace5/1, Out/1
  Mux/1 -> Delay1/1, Flip/1

== system benchmark_ivan_PIANN/SO5_control1/Filter_Prediction1/DAE_MLP2/Sliding Window2 ==
  In : Inport
  Delay1 : Delay  DelayLength=1  InitialCondition=6  SampleTime=t_simulink
  Flip : DSPFlip
  IC : InitialCondition  Value=ic_sw_Snh4
  Mux : Mux  Inputs=2
  To Workspace5 : ToWorkspace  VariableName=sw_Snh4  SampleTime=1/96
  Variable Selector : dspindex/Variable Selector  NumInputs=1  rowsOrCols=Rows  IdxMode=Fixed  Elements=1:(n_sw_inverse-1)  ZerOneIdxMode=One-based  errmode=Clip Index  FillMode=on  FillValues=0
  Out : Outport  VectorParamsAs1DForOutWhenUnconnected=off
  wires:
  IC/1 -> Variable Selector/1
  Delay1/1 -> IC/1
  In/1 -> Mux/1
  Variable Selector/1 -> Mux/2
  Flip/1 -> To Workspace5/1, Out/1
  Mux/1 -> Delay1/1, Flip/1

== system benchmark_ivan_PIANN/SO5_control1/Filter_Prediction1/DAE_MLP2/Sliding Window5 ==
  In : Inport
  Delay1 : Delay  DelayLength=1  InitialCondition=8  SampleTime=t_simulink
  Flip : DSPFlip
  IC : InitialCondition  Value=ic_sw_Sno4
  Mux : Mux  Inputs=2
  To Workspace5 : ToWorkspace  VariableName=sw_Sno4  SampleTime=1/96
  Variable Selector : dspindex/Variable Selector  NumInputs=1  rowsOrCols=Rows  IdxMode=Fixed  Elements=1:(n_sw_inverse-1)  ZerOneIdxMode=One-based  errmode=Clip Index  FillMode=on  FillValues=0
  Out : Outport  VectorParamsAs1DForOutWhenUnconnected=off
  wires:
  IC/1 -> Variable Selector/1
  Delay1/1 -> IC/1
  In/1 -> Mux/1
  Variable Selector/1 -> Mux/2
  Flip/1 -> To Workspace5/1, Out/1
  Mux/1 -> Delay1/1, Flip/1

== system benchmark_ivan_PIANN/SO5_control1/Filter_Prediction1/DAE_MLP2/Sliding Window7 ==
  In : Inport
  Delay1 : Delay  DelayLength=1  InitialCondition=3  SampleTime=t_simulink
  Flip : DSPFlip
  IC : InitialCondition  Value=ic_sw_So4
  Mux : Mux  Inputs=2
  To Workspace5 : ToWorkspace  VariableName=sw_So4  SampleTime=1/96
  Variable Selector : dspindex/Variable Selector  NumInputs=1  rowsOrCols=Rows  IdxMode=Fixed  Elements=1:(n_sw_inverse-1)  ZerOneIdxMode=One-based  errmode=Clip Index  FillMode=on  FillValues=0
  Out : Outport  VectorParamsAs1DForOutWhenUnconnected=off
  wires:
  IC/1 -> Variable Selector/1
  Delay1/1 -> IC/1
  In/1 -> Mux/1
  Variable Selector/1 -> Mux/2
  Flip/1 -> To Workspace5/1, Out/1
  Mux/1 -> Delay1/1, Flip/1

== system benchmark_ivan_PIANN/SO5_control1/Filter_Prediction1/Direct Prediction LSTM4/Sliding Window2 ==
  In : Inport
  Delay1 : Delay  DelayLength=1  InitialCondition=145  SampleTime=t_simulink
  Flip : DSPFlip
  IC : InitialCondition  Value=ic_sw_Kla
  Mux : Mux  Inputs=2
  To Workspace5 : ToWorkspace  VariableName=sw_Kla  SampleTime=1/96
  Variable Selector : dspindex/Variable Selector  NumInputs=1  rowsOrCols=Rows  IdxMode=Fixed  Elements=1:(n_sw_inverse-1)  ZerOneIdxMode=One-based  errmode=Clip Index  FillMode=on  FillValues=0
  Out : Outport  VectorParamsAs1DForOutWhenUnconnected=off
  wires:
  IC/1 -> Variable Selector/1
  Delay1/1 -> IC/1
  In/1 -> Mux/1
  Variable Selector/1 -> Mux/2
  Flip/1 -> To Workspace5/1, Out/1
  Mux/1 -> Delay1/1, Flip/1

== system benchmark_ivan_PIANN/SO5_control_paper/Filter_Prediction/DAE_MLP1/DAE ==
  x_norm : Inport
  Predict RNN : MATLAB Function  TreatAsAtomicUnit=on
  y_n : Outport  VectorParamsAs1DForOutWhenUnconnected=off
  wires:
  Predict RNN/1(prediction) -> y_n/1
  x_norm/1 -> Predict RNN/1(data_in)

== system benchmark_ivan_PIANN/SO5_control_paper/Filter_Prediction/DAE_MLP1/Data Preprocesing Direct ==
  u_n : Inport
  Normalization Values : MATLAB Function  TreatAsAtomicUnit=on
  Out1 : Outport  VectorParamsAs1DForOutWhenUnconnected=off
  wires:
  u_n/1 -> Normalization Values/1(data_input)
  Normalization Values/1(data_norm) -> Out1/1

== system benchmark_ivan_PIANN/SO5_control_paper/Filter_Prediction/DAE_MLP1/Data Preprocessing Direct1 ==
  y_n : Inport
  Denormalization Values : MATLAB Function  TreatAsAtomicUnit=on
  Out1 : Outport  VectorParamsAs1DForOutWhenUnconnected=off
  wires:
  Denormalization Values/1(data_dir) -> Out1/1
  y_n/1 -> Denormalization Values/1(data_input)

== system benchmark_ivan_PIANN/SO5_control_paper/Filter_Prediction/DAE_MLP1/Sliding Window ==
  So4 : Inport
  Sno4 : Inport  Port=2
  Snh4 : Inport  Port=3
  Math Function : Math  Operator=transpose  SignedPower=on
  Matrix Concatenate : Concatenate  NumInputs=3  Mode=Multidimensional array  ConcatenateDimension=2
  Reshape : Reshape  OutputDimensionality=Row vector (2-D)
  Sliding Window3 : Subsystem
  Sliding Window4 : Subsystem
  Sliding Window6 : Subsystem
  Out1 : Outport  VectorParamsAs1DForOutWhenUnconnected=off
  wires:
  Sliding Window6/1(Out) -> Matrix Concatenate/1
  Sliding Window4/1(Out) -> Matrix Concatenate/2
  Sliding Window3/1(Out) -> Matrix Concatenate/3
  So4/1 -> Sliding Window6/1(In)
  Sno4/1 -> Sliding Window4/1(In)
  Snh4/1 -> Sliding Window3/1(In)
  Math Function/1 -> Reshape/1
  Matrix Concatenate/1 -> Math Function/1
  Reshape/1 -> Out1/1

== system benchmark_ivan_PIANN/SO5_control_paper/Filter_Prediction/DAE_MLP2/DAE ==
  x_norm : Inport
  Predict RNN : MATLAB Function  TreatAsAtomicUnit=on
  y_n : Outport  VectorParamsAs1DForOutWhenUnconnected=off
  wires:
  Predict RNN/1(prediction) -> y_n/1
  x_norm/1 -> Predict RNN/1(data_in)

== system benchmark_ivan_PIANN/SO5_control_paper/Filter_Prediction/DAE_MLP2/Data Preprocesing Direct ==
  u_n : Inport
  Normalization Values : MATLAB Function  TreatAsAtomicUnit=on
  Out1 : Outport  VectorParamsAs1DForOutWhenUnconnected=off
  wires:
  u_n/1 -> Normalization Values/1(data_input)
  Normalization Values/1(data_norm) -> Out1/1

== system benchmark_ivan_PIANN/SO5_control_paper/Filter_Prediction/DAE_MLP2/Data Preprocessing Direct1 ==
  y_n : Inport
  Denormalization Values : MATLAB Function  TreatAsAtomicUnit=on
  Out1 : Outport  VectorParamsAs1DForOutWhenUnconnected=off
  wires:
  Denormalization Values/1(data_dir) -> Out1/1
  y_n/1 -> Denormalization Values/1(data_input)

== system benchmark_ivan_PIANN/SO5_control_paper/Filter_Prediction/DAE_MLP2/Sliding Window ==
  So4 : Inport
  Sno4 : Inport  Port=2
  Snh4 : Inport  Port=3
  So5 : Inport  Port=4
  Math Function : Math  Operator=transpose  SignedPower=on
  Matrix Concatenate : Concatenate  NumInputs=4  Mode=Multidimensional array  ConcatenateDimension=2
  Reshape : Reshape  OutputDimensionality=Row vector (2-D)
  Sliding Window1 : Subsystem
  Sliding Window2 : Subsystem
  Sliding Window5 : Subsystem
  Sliding Window7 : Subsystem
  Out1 : Outport  VectorParamsAs1DForOutWhenUnconnected=off
  wires:
  Sliding Window7/1(Out) -> Matrix Concatenate/1
  Sliding Window5/1(Out) -> Matrix Concatenate/2
  Sliding Window2/1(Out) -> Matrix Concatenate/3
  So4/1 -> Sliding Window7/1(In)
  Sno4/1 -> Sliding Window5/1(In)
  Snh4/1 -> Sliding Window2/1(In)
  Math Function/1 -> Reshape/1
  Matrix Concatenate/1 -> Math Function/1
  Reshape/1 -> Out1/1
  So5/1 -> Sliding Window1/1(In)
  Sliding Window1/1(Out) -> Matrix Concatenate/4

== system benchmark_ivan_PIANN/SO5_control_paper/Filter_Prediction/DAE_MLP3/DAE ==
  x_norm : Inport
  Predict RNN : MATLAB Function  TreatAsAtomicUnit=on
  y_n : Outport  VectorParamsAs1DForOutWhenUnconnected=off
  wires:
  Predict RNN/1(prediction) -> y_n/1
  x_norm/1 -> Predict RNN/1(data_in)

== system benchmark_ivan_PIANN/SO5_control_paper/Filter_Prediction/DAE_MLP3/Data Preprocesing Direct ==
  u_n : Inport
  Normalization Values : MATLAB Function  TreatAsAtomicUnit=on
  Out1 : Outport  VectorParamsAs1DForOutWhenUnconnected=off
  wires:
  u_n/1 -> Normalization Values/1(data_input)
  Normalization Values/1(data_norm) -> Out1/1

== system benchmark_ivan_PIANN/SO5_control_paper/Filter_Prediction/DAE_MLP3/Data Preprocessing Direct1 ==
  y_n : Inport
  Denormalization Values : MATLAB Function  TreatAsAtomicUnit=on
  Out1 : Outport  VectorParamsAs1DForOutWhenUnconnected=off
  wires:
  Denormalization Values/1(data_dir) -> Out1/1
  y_n/1 -> Denormalization Values/1(data_input)

== system benchmark_ivan_PIANN/SO5_control_paper/Filter_Prediction/DAE_MLP3/Sliding Window ==
  Snh4 : Inport
  So5 : Inport  Port=2
  TSS4 : Inport  Port=3
  Q4 : Inport  Port=4
  Math Function : Math  Operator=transpose  SignedPower=on
  Matrix Concatenate : Concatenate  NumInputs=4  Mode=Multidimensional array  ConcatenateDimension=2
  Reshape : Reshape  OutputDimensionality=Row vector (2-D)
  Sliding Window Buffer Snh4 : Subsystem
  Sliding Window Buffer Sno4 : Subsystem
  Sliding Window Buffer So4 : Subsystem
  Sliding Window Buffer So5 : Subsystem
  Sliding Window1 : Subsystem  Commented=on
  Sliding Window2 : Subsystem  Commented=on
  Sliding Window5 : Subsystem  Commented=on
  Sliding Window7 : Subsystem  Commented=on
  Out1 : Outport  VectorParamsAs1DForOutWhenUnconnected=off
  wires:
  Sliding Window Buffer Snh4/1(Out1) -> Matrix Concatenate/1
  Sliding Window Buffer So5/1(Out1) -> Matrix Concatenate/2
  Sliding Window Buffer So4/1(Out1) -> Matrix Concatenate/3
  Snh4/1 -> Sliding Window Buffer Snh4/1(In1)
  So5/1 -> Sliding Window Buffer So5/1(In1)
  TSS4/1 -> Sliding Window Buffer So4/1(In1)
  Math Function/1 -> Reshape/1
  Matrix Concatenate/1 -> Math Function/1
  Reshape/1 -> Out1/1
  Q4/1 -> Sliding Window Buffer Sno4/1(In1)
  Sliding Window Buffer Sno4/1(Out1) -> Matrix Concatenate/4

== system benchmark_ivan_PIANN/SO5_control_paper/Filter_Prediction/DAE_lstm/DAE ==
  x_norm : Inport
  Predict RNN : MATLAB Function  TreatAsAtomicUnit=on
  y_n : Outport  VectorParamsAs1DForOutWhenUnconnected=off
  wires:
  Predict RNN/1(prediction) -> y_n/1
  x_norm/1 -> Predict RNN/1(data_in)

== system benchmark_ivan_PIANN/SO5_control_paper/Filter_Prediction/DAE_lstm/Data Preprocesing Direct ==
  u_n : Inport
  Math Function : Math  Operator=transpose  SignedPower=on
  Normalizer1 : Subsystem
  Reshape : Reshape  OutputDimensionality=Row vector (2-D)
  Out1 : Outport  VectorParamsAs1DForOutWhenUnconnected=off
  wires:
  Reshape/1 -> Out1/1
  Normalizer1/1(Data Normalized) -> Math Function/1
  Math Function/1 -> Reshape/1
  u_n/1 -> Normalizer1/1(Data Input)
